simulink model "DC_motor"  (R2024a)
settings: Solver=VariableStepAuto  StartTime=0.0  StopTime=10.0  RelTol=1e-3
values from neighbouring files (symbols this model uses):
  drivetrain_gain = 10.5    [assignment_2.m]
  J_motor = (2 * Ir * (1 / drivetrain_gain^2))    (= 0.026485260771)    [assignment_2.m]
  K_b = K_m    (= 0.185017621344)    [assignment_2.m]
  K_m = T_max / omega_max_rad    (= 0.185017621344)    [assignment_2.m]
  L_motor = tau_m * R_motor    (= 0.125)    [assignment_2.m]
  motor_eff = 0.9    [assignment_2.m]
  R = 0.3488    [assignment_2.m]
  R_motor = 2.5    [assignment_2.m]
  velstart = 20    [assignment_2.m]
settings Model: Creator=fjmo  LastModifiedBy=fjmo

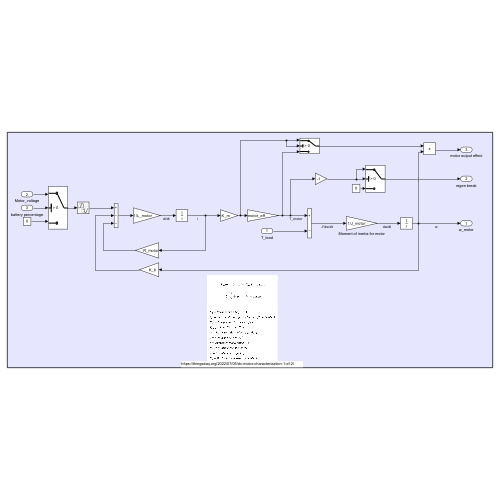
[thumbnail: Simulink's stored preview of the top-level diagram]
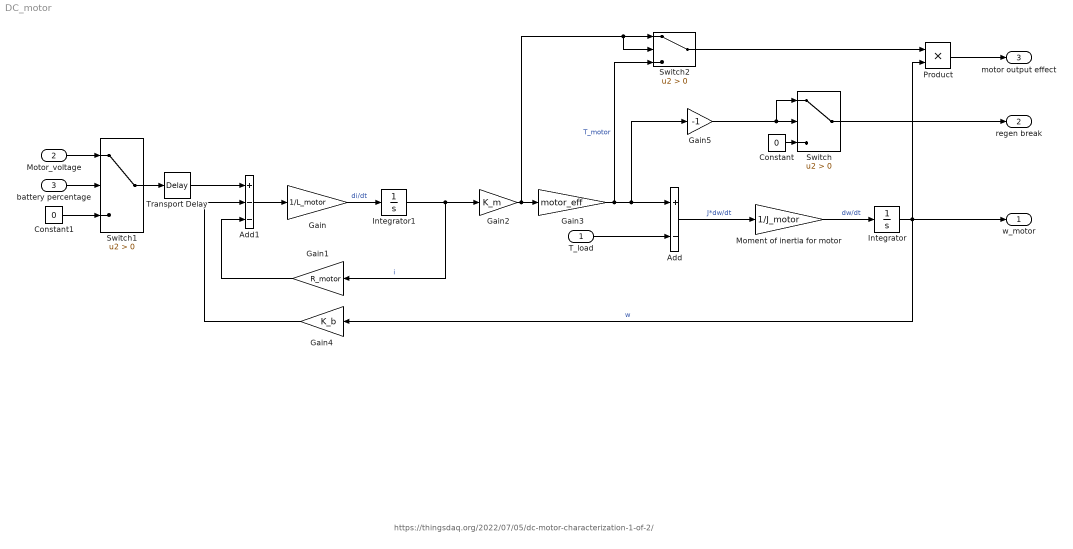
== system DC_motor ==
  note: https://thingsdaq.org/2022/07/05/dc-motor-characterization-1-of-2/
  T_load : Inport
  Motor_voltage : Inport  Port=2
  battery percentage : Inport  Port=3
  Add : Sum  Inputs=+-
  Add1 : Sum  Inputs=+--
  Constant : Constant  Value=0
  Constant1 : Constant  Value=0
  Gain : Gain  Gain=1/L_motor
  Gain1 : Gain  Gain=R_motor
  Gain2 : Gain  Gain=K_m
  Gain3 : Gain  Gain=motor_eff
  Gain4 : Gain  Gain=K_b
  Gain5 : Gain  Gain=-1
  Integrator : Integrator  InitialCondition=velstart/R*drivetrain_gain
  Integrator1 : Integrator
  Moment of inertia for motor : Gain  Gain=1/J_motor
  Product : Product
  Switch : Switch  Criteria=u2 > Threshold  SaturateOnIntegerOverflow=off  InputSameDT=off
  Switch1 : Switch  Criteria=u2 > Threshold  SaturateOnIntegerOverflow=off  InputSameDT=off
  Switch2 : Switch  Criteria=u2 > Threshold  SaturateOnIntegerOverflow=off  InputSameDT=off
  Transport Delay : TransportDelay  DelayTime=20*10^(-3)
  w_motor : Outport
  regen break : Outport  Port=2
  motor output effect : Outport  Port=3
  wires:
  Moment of inertia for motor/1 -> Integrator/1  "dw/dt"
  Add/1 -> Moment of inertia for motor/1  "J*dw/dt"
  Integrator/1 -> Product/2, w_motor/1, Gain4/1  "w"
  Integrator1/1 -> Gain2/1, Gain1/1  "i"
  Gain/1 -> Integrator1/1  "di/dt"
  Add1/1 -> Gain/1
  Gain2/1 -> Switch2/2, Switch2/1, Gain3/1
  Gain3/1 -> Switch2/3, Gain5/1, Add/1  "T_motor"
  T_load/1 -> Add/2
  Gain1/1 -> Add1/3
  Gain4/1 -> Add1/2
  Gain5/1 -> Switch/1, Switch/2
  Constant/1 -> Switch/3
  Switch/1 -> regen break/1
  Motor_voltage/1 -> Switch1/1
  battery percentage/1 -> Switch1/2
  Constant1/1 -> Switch1/3
  Product/1 -> motor output effect/1
  Switch2/1 -> Product/1
  Switch1/1 -> Transport Delay/1
  Transport Delay/1 -> Add1/1
